simulink model "ramp_test"  (R2021a)
settings: Solver=VariableStepAuto  StartTime=0.0  StopTime=10  RelTol=1e-3
libraries: simulink x1
settings Model: SimulationMode=accelerator  Creator=tejal  LastModifiedBy=dhruv
settings SolverCC: ZeroCrossAlgorithm=Adaptive
settings DebuggingCC: IgnoredZcDiagnostic=none

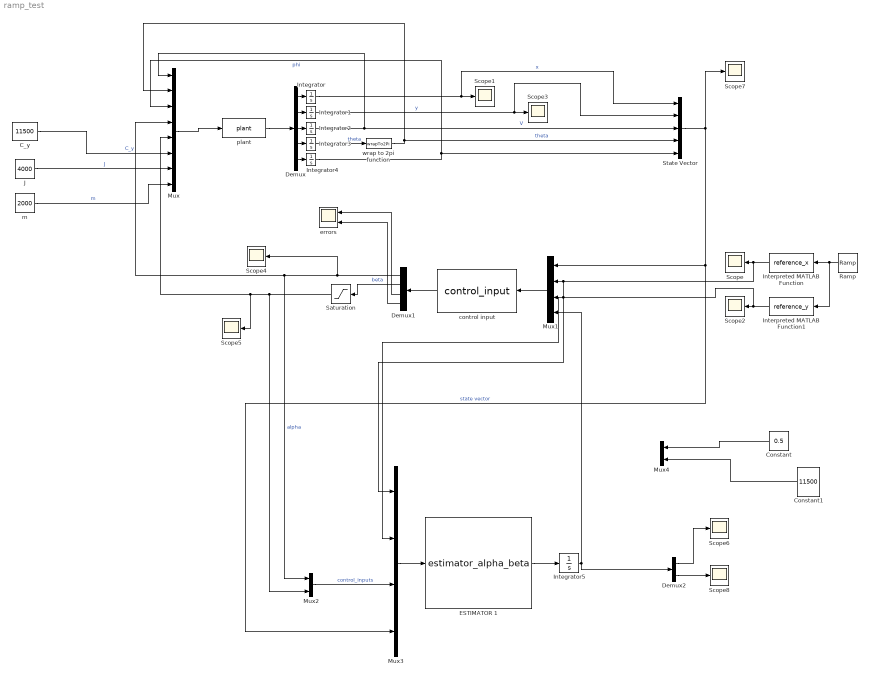
== system ramp_test ==
  C_y : Constant  Value=11500
  Constant : Constant  Value=0.5
  Constant1 : Constant  Value=11500
  Demux : Demux  Outputs=5
  Demux1 : Demux
  Demux2 : Demux  Outputs=2
  ESTIMATOR 1 : MATLABFcn  MATLABFcn=estimator_alpha_beta  OutputDimensions=2
  Integrator : Integrator  InitialCondition=0.0005
  Integrator1 : Integrator  InitialCondition=0.00005
  Integrator2 : Integrator  InitialCondition=10  UpperSaturationLimit=100  LowerSaturationLimit=-10
  Integrator3 : Integrator  InitialCondition=0.7
  Integrator4 : Integrator  UpperSaturationLimit=100  LowerSaturationLimit=-100
  Integrator5 : Integrator  InitialCondition=[0.4;11000]
  Interpreted MATLAB Function : MATLABFcn  MATLABFcn=reference_x  OutputDimensions=4
  Interpreted MATLAB Function1 : MATLABFcn  MATLABFcn=reference_y  OutputDimensions=4
  J : Constant  Value=4000
  Mux : Mux  Inputs=8
  Mux1 : Mux
  Mux2 : Mux  Inputs=2
  Mux3 : Mux
  Mux4 : Mux  Inputs=2
  Ramp : simulink/Sources/Ramp  slope=10  start=0  InitialOutput=0
  Saturation : Saturate  UpperLimit=25  LowerLimit=-25
  Scope{,1..8} (9 alike) : Scope
  State Vector : Mux  Inputs=5
  control input : MATLABFcn  MATLABFcn=control_input  OutputDimensions=4
  errors : Scope  NumInputPorts=2
  m : Constant  Value=2000
  plant : MATLABFcn  MATLABFcn=plant  OutputDimensions=5
  wrap to 2pi function : MATLABFcn  MATLABFcn=wrapTo2Pi
  wires:
  Mux/1 -> plant/1
  plant/1 -> Demux/1
  Demux/1 -> Integrator/1
  Demux/5 -> Integrator4/1
  Demux/4 -> Integrator3/1
  Demux/3 -> Integrator2/1
  Demux/2 -> Integrator1/1
  Integrator/1 -> State Vector/1, Scope1/1  "x"
  Integrator1/1 -> State Vector/2, Scope3/1  "y"
  Integrator2/1 -> Mux/1, State Vector/3  "V"
  Integrator3/1 -> wrap to 2pi function/1  "theta"
  Integrator4/1 -> State Vector/5, Mux/3  "phi"
  J/1 -> Mux/7  "J"
  control input/1 -> Demux1/1
  Mux1/1 -> control input/1
  wrap to 2pi function/1 -> State Vector/4, Mux/2  "theta"
  Demux1/3 -> errors/1
  Demux1/4 -> errors/2
  C_y/1 -> Mux/6  "C_y"
  Demux1/2 -> Saturation/1  "beta"
  Demux1/1 -> Mux/4, Mux2/1, Scope4/1  "alpha"
  m/1 -> Mux/8  "m"
  State Vector/1 -> Mux3/4, Mux1/1, Scope7/1  "state vector"
  Mux3/1 -> ESTIMATOR 1/1
  ESTIMATOR 1/1 -> Integrator5/1
  Integrator5/1 -> Mux1/4, Demux2/1
  Mux2/1 -> Mux3/3  "control_inputs"
  Demux2/2 -> Scope8/1
  Demux2/1 -> Scope6/1
  Constant/1 -> Mux4/1
  Constant1/1 -> Mux4/2
  Ramp/1 -> Interpreted MATLAB Function1/1, Interpreted MATLAB Function/1
  Interpreted MATLAB Function/1 -> Mux3/1, Mux1/2, Scope/1
  Interpreted MATLAB Function1/1 -> Mux3/2, Mux1/3, Scope2/1
  Saturation/1 -> Mux2/2, Scope5/1, Mux/5
